simulink model "VSI_IM"  (Simulink 7.3)
settings: Solver=ode45  StartTime=0.0  StopTime=1  RelTol=1e-3
libraries: powerlib x9
settings Model: Creator=Debmalya Mukherjee  LastModifiedBy=Debmalya Mukherjee

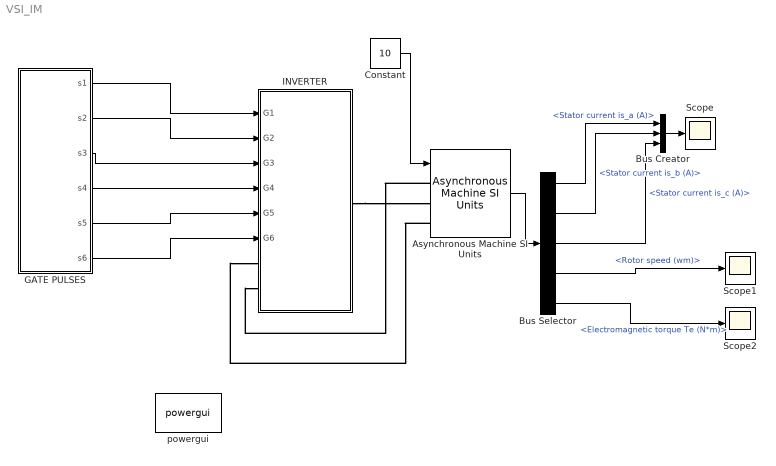
== system VSI_IM ==
  Asynchronous Machine SI Units : powerlib/Machines/Asynchronous Machine SI Units  DialogController=POWERSYS.PowerSysDialog  SystemSampleTime=-1  PresetModel=No  MechanicalLoad=Torque Tm  ShowDetailedParameters=on  RotorType=Squirrel-cage  ReferenceFrame=Rotor  NominalParameters=[10422.6 415 50]  Stator=[1.09 .006]  Rotor=[1.09 .006]  Lm=.072  Mechanical=[.1 .03 2]  PolePairs=2  InitialConditions=[1 0 0 0 0 0 0 0]  Units=SI  LoadFlowParameters=1492000  SimulateSaturation=off  Saturation=[14.03593122, 27.81365428, 53.79336849, 72.68890987, 97.98006896, 148.6815601, 215.7428561, 302.9841135, 428.7778367 ; 230, 322, 414, 460, 506, 552, 598, 644, 690]  TsPowergui=0  TsBlock=-1  IterativeModel=Forward Euler
  Bus Creator : BusCreator  Inputs=3
  Bus Selector : BusSelector  OutputSignals=Stator measurements.Stator current is_a (A),Stator measurements.Stator current is_b (A),Stator measurements.Stator current is_c (A),Mechanical.Rotor speed (wm),Mechanical.Electromagnetic torque Te (N*m)
  Constant : Constant  Value=10  OutDataType=fixdt(1, 16)  OutScaling=2^0
  GATE PULSES : Subsystem
  INVERTER : Subsystem
  Scope : Scope
  Scope1 : Scope
      settings: TimeRange=0.07000000000000001  YMin=-47  YMax=-40
  Scope2 : Scope
      settings: SaveName=ScopeData2
  powergui : powerlib/powergui  Priority=1  SystemSampleTime=-1  SimulationMode=Continuous  SampleTime=50e-6  frequency=50  SPID=off  DisableSnubberDevices=off  DisableRonSwitches=off  DisableVfSwitches=off  SwTol=0  Interpol=off  frequencyindice=50  echomessages=off  HookPort=off  DisplayEquations=off  FunctionMessages=off  EnableUseOfTLC=off  x0status=blocks  RestoreLinks=warning  Frange=[0:2:500]  Ylog=off  Xlog=on  ShowGrid=off  save=off  variable=ZData  ZoomFFT=on  StartTime=0.0  cycles=1  DisplayStyle=1  fundamental=60  FreqAxis=off  MaxFrequency=1000  frequencyindicesteady=1  RmsSteady=1  display=off  Ts=0  methode=off
  wires:
  GATE PULSES/1(s1) -> INVERTER/1(G1)
  GATE PULSES/2(s2) -> INVERTER/2(G2)
  GATE PULSES/3(s3) -> INVERTER/3(G3)
  GATE PULSES/4(s4) -> INVERTER/4(G4)
  GATE PULSES/5(s5) -> INVERTER/5(G5)
  GATE PULSES/6(s6) -> INVERTER/6(G6)
  Constant/1 -> Asynchronous Machine SI Units/1
  Asynchronous Machine SI Units/1 -> Bus Selector/1
  Bus Creator/1 -> Scope/1
  Bus Selector/1 -> Bus Creator/1  "<Stator current is_a (A)>"
  Bus Selector/3 -> Bus Creator/3  "<Stator current is_c (A)>"
  Bus Selector/2 -> Bus Creator/2  "<Stator current is_b (A)>"
  Bus Selector/4 -> Scope1/1  "<Rotor speed (wm)>"
  Bus Selector/5 -> Scope2/1  "<Electromagnetic torque Te (N*m)>"
  connections:
  INVERTER/RConn1 -- Asynchronous Machine SI Units/LConn2
  Asynchronous Machine SI Units/LConn1 -- INVERTER/LConn2
  Asynchronous Machine SI Units/LConn3 -- INVERTER/LConn1

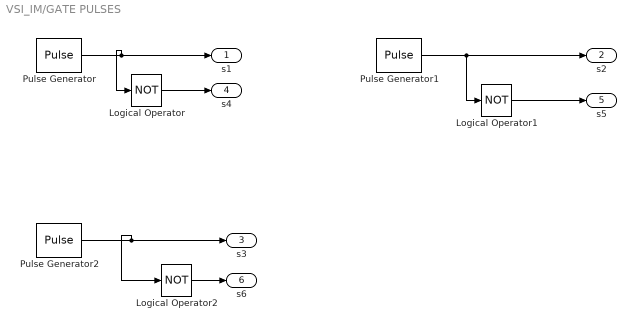
== system VSI_IM/GATE PULSES ==
  Logical Operator : Logic  Operator=NOT  AllPortsSameDT=off  OutDataTypeMode=boolean  LogicDataType=fixdt(0, 8)  OutDataTypeStr=boolean
  Logical Operator1 : Logic  Operator=NOT  AllPortsSameDT=off  OutDataTypeMode=boolean  LogicDataType=fixdt(0, 8)  OutDataTypeStr=boolean
  Logical Operator2 : Logic  Operator=NOT  AllPortsSameDT=off  OutDataTypeMode=boolean  LogicDataType=fixdt(0, 8)  OutDataTypeStr=boolean
  Pulse Generator : DiscretePulseGenerator  PulseType=Time based  Amplitude=1  Period=.02  PulseWidth=50  PhaseDelay=0  SampleTime=1
  Pulse Generator1 : DiscretePulseGenerator  PulseType=Time based  Amplitude=1  Period=.02  PulseWidth=50  PhaseDelay=0.0033  SampleTime=1
  Pulse Generator2 : DiscretePulseGenerator  PulseType=Time based  Amplitude=1  Period=.02  PulseWidth=50  PhaseDelay=0.0067  SampleTime=1
  s1 : Outport  OutDataType=fixdt(1, 16)  OutScaling=2^0
  s2 : Outport  Port=2  OutDataType=fixdt(1, 16)  OutScaling=2^0
  s3 : Outport  Port=3  OutDataType=fixdt(1, 16)  OutScaling=2^0
  s4 : Outport  Port=4  OutDataType=fixdt(1, 16)  OutScaling=2^0
  s5 : Outport  Port=5  OutDataType=fixdt(1, 16)  OutScaling=2^0
  s6 : Outport  Port=6  OutDataType=fixdt(1, 16)  OutScaling=2^0
  wires:
  Pulse Generator/1 -> s1/1, Logical Operator/1
  Pulse Generator1/1 -> s2/1, Logical Operator1/1
  Pulse Generator2/1 -> s3/1, Logical Operator2/1
  Logical Operator/1 -> s4/1
  Logical Operator1/1 -> s5/1
  Logical Operator2/1 -> s6/1

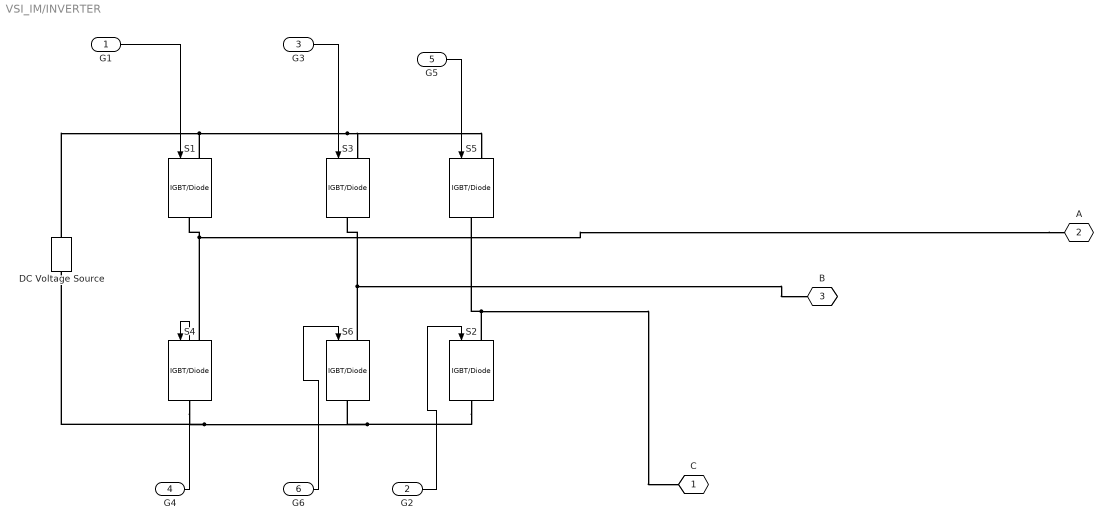
== system VSI_IM/INVERTER ==
  G1 : Inport  OutDataType=fixdt(1, 16)  OutScaling=2^0
  G2 : Inport  Port=2  OutDataType=fixdt(1, 16)  OutScaling=2^0
  G3 : Inport  Port=3  OutDataType=fixdt(1, 16)  OutScaling=2^0
  G4 : Inport  Port=4  OutDataType=fixdt(1, 16)  OutScaling=2^0
  G5 : Inport  Port=5  OutDataType=fixdt(1, 16)  OutScaling=2^0
  G6 : Inport  Port=6  OutDataType=fixdt(1, 16)  OutScaling=2^0
  DC Voltage Source : powerlib/Electrical Sources/DC Voltage Source  DialogController=POWERSYS.PowerSysDialog  SystemSampleTime=-1  Amplitude=600  Measurements=None
  S{1..6} (6 alike) : powerlib/Power Electronics/IGBT//Diode  DialogController=POWERSYS.PowerSysDialog  SystemSampleTime=-1  Ron=1e-3  Rs=1e5  Cs=inf  Measurements=off
  C : PMIOPort  Tag=PMCPort  Port=1  Side=Left
  A : PMIOPort  Tag=PMCPort  Port=2  Side=Left
  B : PMIOPort  Tag=PMCPort  Port=3  Side=Right
  wires:
  G1/1 -> S1/1
  G2/1 -> S2/1
  G3/1 -> S3/1
  G4/1 -> S4/1
  G5/1 -> S5/1
  G6/1 -> S6/1
  connections:
  S2/RConn1 -- S6/RConn1 -- DC Voltage Source/LConn1 -- S4/RConn1
  DC Voltage Source/RConn1 -- S1/LConn1 -- S3/LConn1 -- S5/LConn1
  S6/LConn1 -- S3/RConn1 -- B/RConn1
  A/RConn1 -- S4/LConn1 -- S1/RConn1
  S2/LConn1 -- S5/RConn1 -- C/RConn1
